simulink model "signal_generator"  (R2016b)
settings: Solver=VariableStepAuto  StartTime=0.0  StopTime=0.5  RelTol=1e-3
libraries: commutil2 x1
settings Model: Creator=张尧  LastModifiedBy=张尧

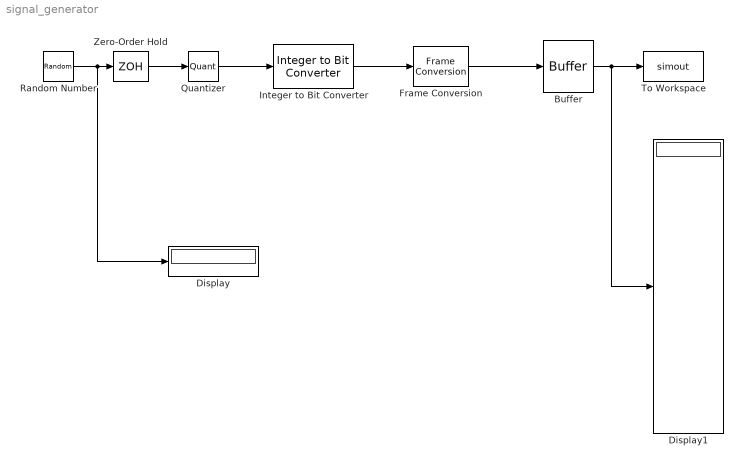
== system signal_generator ==
  Buffer : Buffer  N=16  TreatMby1Signals=One channel  OutputFrames=off
  Display : Display
  Display1 : Display
      settings: Decimation=8
  Frame Conversion : FrameConversion  InheritSamplingMode=off
  Integer to Bit Converter : commutil2/Integer to Bit Converter  nbits=16  signedInputValues=Unsigned  bitOrder=MSB first  outDtype=double
  Quantizer : Quantizer  QuantizationInterval=1
  Random Number : RandomNumber  Mean=32768  Variance=100  Seed=20  SampleTime=20
  To Workspace : ToWorkspace  VariableName=simout  SampleTime=-1
      settings: Save2DSignal=2-D array (concatenate along first dimension)
  Zero-Order Hold : ZeroOrderHold
  wires:
  Zero-Order Hold/1 -> Quantizer/1
  Quantizer/1 -> Integer to Bit Converter/1
  Integer to Bit Converter/1 -> Frame Conversion/1
  Frame Conversion/1 -> Buffer/1
  Random Number/1 -> Display/1, Zero-Order Hold/1
  Buffer/1 -> To Workspace/1, Display1/1
